simulink model "PowerSplitDriveUnitBasic_test_harness"  (R2020b)
settings: Solver=VariableStepAuto  StartTime=0.0  StopTime=t_end  RelTol=1e-3  AbsTol=1e-3
PreLoadFcn:
  | PowerSplitDriveUnitBasic_setup
undefined symbols (not defined in the file or in its folder): testharness
libraries: fl_lib x1, nesl_utility x1, EVComponents_utility_lib x1
settings Model: Creator=isaacito  LastModifiedBy=isaacito
settings SolverCC: AutoScaleAbsTol=off
settings DataIOCC: DSMLogging=off  InspectSignalLogs=on
settings SimscapeCC: SimscapeLogType=all  SimscapeLogSimulationStatistics=on  SimscapeLogLimitData=off

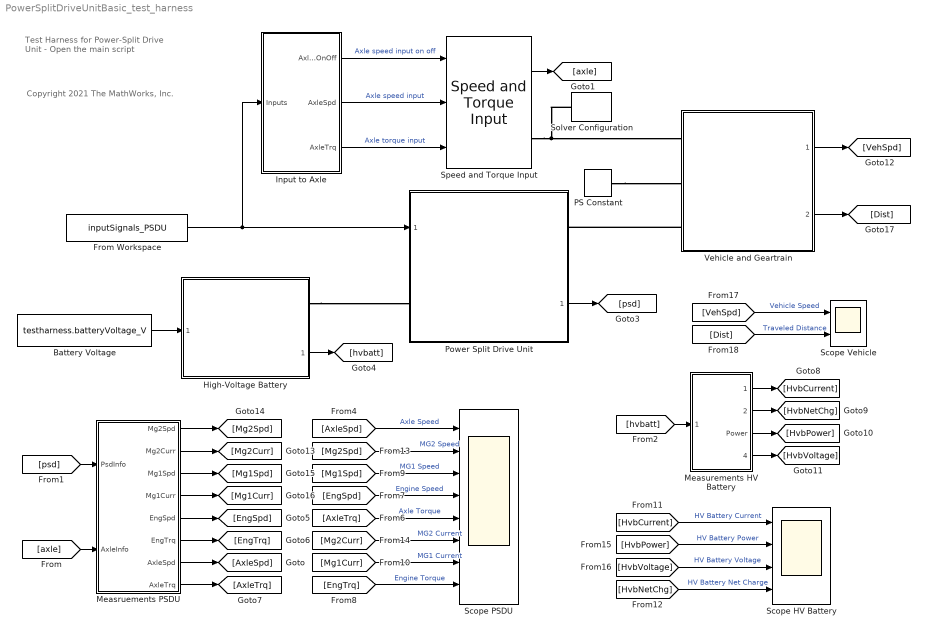
== system PowerSplitDriveUnitBasic_test_harness ==
  note: Copyright 2021 The MathWorks, Inc.
  note: Test Harness for
      | Power-Split Drive Unit
      | - Open the main script
  Battery Voltage : Constant  Value=testharness.batteryVoltage_V
  From Workspace : FromWorkspace  VariableName=inputSignals_PSDU  OutDataTypeStr=Bus: inputBus_PSDU  Interpolate=off  OutputAfterFinalValue=Holding final value
      settings: AttributesFormatString=%<OutDataTypeStr>
  High-Voltage Battery : Subsystem  ReferencedSubsystem=BatteryForTest_refsub
      settings: PortSchema="{\"entries\":[{\"content\":{\"sides\":[{\"content\":{\"connectorIds\":[\"In1\"]},\"type\":\"ConnectorPlacement.EquallySpacedRectSide\",\"uuid\":\"6ec42dc2-af13-403d-bb44-bbfe17049ebb\"},{\"content\":{\"connectorIds\":[\"RConn1\",\"Out1\"],\"side\":\"RIGHT\"},\"type\":\"ConnectorPlacement.EquallySpacedRectSide\",\"uuid\":\"18b43a22-b216-415c-b9ff-5dd426481655\"},{\"content\":{\"connectorIds\":[],\"side\":\"TOP\"},\"type\":\"ConnectorPlacement.EquallySpacedRectSide\",\"uuid\":\"9ddf6635-2c27-427a-8c83-df626a0e9ed3\"},{\"content\":{\"connectorIds\":[],\"side\":\"HIDDEN\"},\"type\":\"ConnectorPlacement.EquallySpacedRectSide\",\"uuid\":\"332981be-c8a8-46f3-86be-153015cc7779\"}]},\"type\":\"ConnectorPlacement.EquallySpacedConnector\",\"uuid\":\"0a64d723-305c-452f-a915-e14881ea19f7\"}],\"packageUris\":[\"http://schema.mathworks.com/mf0/Connector/R2020b\"],\"version\":\"1.0\"}"
  Input to Axle : Subsystem
  Measruements PSDU : Subsystem
  Measurements HV Battery : Subsystem
  PS Constant : fl_lib/Physical Signals/Sources/PS Constant  constant=0 N
      settings: AttributesFormatString=%<constant> [%<constant_unit>]
  Power Split Drive Unit : Subsystem  ReferencedSubsystem=PowerSplitDriveUnitBasic_refsub
      settings: PortSchema="{\"entries\":[{\"content\":{\"sides\":[{\"content\":{\"connectorIds\":[\"In1\",\"LConn1\"]},\"type\":\"ConnectorPlacement.EquallySpacedRectSide\",\"uuid\":\"ac3719a4-f5ca-49c1-b88d-60ddfcbc9c3c\"},{\"content\":{\"connectorIds\":[\"RConn1\",\"Out1\"],\"side\":\"RIGHT\"},\"type\":\"ConnectorPlacement.EquallySpacedRectSide\",\"uuid\":\"02c1cdca-c4bc-4e36-8da7-b9fd13165580\"},{\"content\":{\"connectorIds\":[],\"side\":\"TOP\"},\"type\":\"ConnectorPlacement.EquallySpacedRectSide\",\"uuid\":\"9a293679-982e-42e0-b445-a53b2f9deeb2\"},{\"content\":{\"connectorIds\":[],\"side\":\"HIDDEN\"},\"type\":\"ConnectorPlacement.EquallySpacedRectSide\",\"uuid\":\"92624000-5028-4c46-b75d-fdf82f03c691\"}]},\"type\":\"ConnectorPlacement.EquallySpacedConnector\",\"uuid\":\"49b414d9-6436-4fd3-904c-291d56adec0c\"}],\"packageUris\":[\"http://schema.mathworks.com/mf0/Connector/R2020b\"],\"version\":\"1.0\"}"
  Scope HV Battery : Scope  NumInputPorts=4
  Scope PSDU : Scope  NumInputPorts=8
  Scope Vehicle : Scope  NumInputPorts=2
  Solver Configuration : nesl_utility/Solver Configuration  PhysicalDomain=network_engine_domain  SubClassName=solver  LeftPortType=input  RightPortType=generic  Tones=[]  Harmonics=[]  SimulateNoise=off  Profile=off  UseLocalSampling=off  EnableSwitchedLinearOptims=on  FrequencyDomain=off  UseCCode=off  RelTol=0.001  AbsTol=1e-06  MinStep=1e-09  ToWorkspace=off  RevertToSquareIcSolve=off  NumHomotopyIterations=100  PhasorMode=off  PhasorModeNumHarmonics=1  DoDC=off  ResidualTolerance=1e-09  UseLocalSolver=off  LocalSolverChoice=NE_BACKWARD_EULER_ADVANCER  LocalSolverSampleTime=0.001  DoFixedCost=off  MaxNonlinIter=3  MaxModeIter=2  ComputeImpulses=off  ImpulseIterations=2  LinearAlgebra=auto  EquationFormulation=NE_TIME_EF  DelaysMemoryBudget=1024  AutomaticFiltering=on  FilteringTimeConstant=0.001  PartitionStorageMethod=AS_NEEDED  PartitionMemoryBudget=1024  PartitionMethod=ROBUST
      settings: AttributesFormatString=Local sover: %<UseLocalSolver>
  Speed and Torque Input : EVComponents_utility_lib/Speed and Torque Input  t_friction=10000  t_locked=10000  w_tol=0.001  initial_state_locked=sdl.enum.initial_lock.unlocked
  Vehicle and Geartrain : Subsystem  ReferencedSubsystem=VehicleForTest_refsub
      settings: PortSchema="{\"entries\":[{\"content\":{\"sides\":[{\"content\":{\"connectorIds\":[\"LConn1\",\"LConn3\",\"LConn2\"]},\"type\":\"ConnectorPlacement.EquallySpacedRectSide\",\"uuid\":\"c975ecd5-3624-4c19-9a80-acedd8bc41a3\"},{\"content\":{\"connectorIds\":[\"Out1\",\"Out2\"],\"side\":\"RIGHT\"},\"type\":\"ConnectorPlacement.EquallySpacedRectSide\",\"uuid\":\"910143c3-3967-4448-a629-d08cf6777789\"},{\"content\":{\"connectorIds\":[],\"side\":\"TOP\"},\"type\":\"ConnectorPlacement.EquallySpacedRectSide\",\"uuid\":\"7a417a30-364f-4b70-8ba2-82e05b7f8ad5\"},{\"content\":{\"connectorIds\":[],\"side\":\"HIDDEN\"},\"type\":\"ConnectorPlacement.EquallySpacedRectSide\",\"uuid\":\"66b5b01a-20fa-4f6a-8c11-38a64c540bf5\"}]},\"type\":\"ConnectorPlacement.EquallySpacedConnector\",\"uuid\":\"d97c4709-181f-4fdd-bd6d-fe96f1a8d0ed\"}],\"packageUris\":[\"http://schema.mathworks.com/mf0/Connector/R2020b\"],\"version\":\"1.0\"}"
  wires:
  Battery Voltage/1 -> High-Voltage Battery/1
  Input to Axle/2(AxleSpd) -> Speed and Torque Input/2  "Axle speed input"
  Input to Axle/1(AxleSpd_OnOff) -> Speed and Torque Input/1  "Axle speed input on off"
  Input to Axle/3(AxleTrq) -> Speed and Torque Input/3  "Axle torque input"
  From Workspace/1 -> Power Split Drive Unit/1, Input to Axle/1(Inputs)
  Speed and Torque Input/1 -> [axle]
  Power Split Drive Unit/1 -> [psd]
  [axle] -> Measruements PSDU/2(AxleInfo)
  [psd] -> Measruements PSDU/1(PsdInfo)
  [EngTrq] -> Scope PSDU/8  "Engine Torque"
  [Mg1Curr] -> Scope PSDU/7  "MG1 Current"
  [EngSpd] -> Scope PSDU/4  "Engine Speed"
  [Mg1Spd] -> Scope PSDU/3  "MG1 Speed"
  [AxleSpd] -> Scope PSDU/1  "Axle Speed"
  [AxleTrq] -> Scope PSDU/5  "Axle Torque"
  [Mg2Curr] -> Scope PSDU/6  "MG2 Current"
  [Mg2Spd] -> Scope PSDU/2  "MG2 Speed"
  Measruements PSDU/1(Mg2Spd) -> [Mg2Spd]
  Measruements PSDU/2(Mg2Curr) -> [Mg2Curr]
  Measruements PSDU/3(Mg1Spd) -> [Mg1Spd]
  Measruements PSDU/4(Mg1Curr) -> [Mg1Curr]
  Measruements PSDU/5(EngSpd) -> [EngSpd]
  Measruements PSDU/6(EngTrq) -> [EngTrq]
  Measruements PSDU/7(AxleSpd) -> [AxleSpd]
  Measruements PSDU/8(AxleTrq) -> [AxleTrq]
  [hvbatt] -> Measurements HV Battery/1(HVBatt)
  [HvbPower] -> Scope HV Battery/2  "HV Battery Power"
  [HvbNetChg] -> Scope HV Battery/4  "HV Battery Net Charge"
  [HvbVoltage] -> Scope HV Battery/3  "HV Battery Voltage"
  [HvbCurrent] -> Scope HV Battery/1  "HV Battery Current"
  Measurements HV Battery/1(Current) -> [HvbCurrent]
  Measurements HV Battery/2(NetChg) -> [HvbNetChg]
  Measurements HV Battery/3(Power) -> [HvbPower]
  Measurements HV Battery/4(Voltage) -> [HvbVoltage]
  Vehicle and Geartrain/1 -> [VehSpd]
  Vehicle and Geartrain/2 -> [Dist]
  [VehSpd] -> Scope Vehicle/1  "Vehicle Speed"
  [Dist] -> Scope Vehicle/2  "Traveled Distance"
  High-Voltage Battery/1 -> [hvbatt]
  connections:
  Vehicle and Geartrain/LConn2 -- Power Split Drive Unit/RConn1
  Speed and Torque Input/RConn1 -- Vehicle and Geartrain/LConn1 -- Solver Configuration/RConn1
  PS Constant/RConn1 -- Vehicle and Geartrain/LConn3
  High-Voltage Battery/RConn1 -- Power Split Drive Unit/LConn1

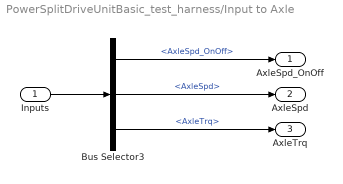
== system PowerSplitDriveUnitBasic_test_harness/Input to Axle ==
  Inputs : Inport
  Bus Selector3 : BusSelector  OutputSignals=AxleSpd_OnOff,AxleSpd,AxleTrq
  AxleSpd_OnOff : Outport
  AxleSpd : Outport  Port=2
  AxleTrq : Outport  Port=3
  wires:
  Bus Selector3/2 -> AxleSpd/1  "<AxleSpd>"
  Inputs/1 -> Bus Selector3/1
  Bus Selector3/1 -> AxleSpd_OnOff/1  "<AxleSpd_OnOff>"
  Bus Selector3/3 -> AxleTrq/1  "<AxleTrq>"

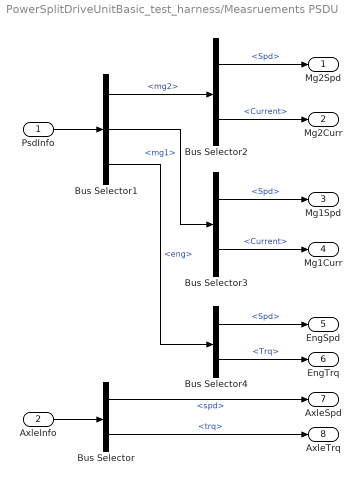
== system PowerSplitDriveUnitBasic_test_harness/Measruements PSDU ==
  PsdInfo : Inport
  AxleInfo : Inport  Port=2
  Bus Selector : BusSelector  OutputSignals=spd,trq
  Bus Selector1 : BusSelector  OutputSignals=mg2,mg1,eng
  Bus Selector2 : BusSelector  OutputSignals=Spd,Current
  Bus Selector3 : BusSelector  OutputSignals=Spd,Current
  Bus Selector4 : BusSelector  OutputSignals=Spd,Trq
  Mg2Spd : Outport
  Mg2Curr : Outport  Port=2
  Mg1Spd : Outport  Port=3
  Mg1Curr : Outport  Port=4
  EngSpd : Outport  Port=5
  EngTrq : Outport  Port=6
  AxleSpd : Outport  Port=7
  AxleTrq : Outport  Port=8
  wires:
  AxleInfo/1 -> Bus Selector/1
  PsdInfo/1 -> Bus Selector1/1
  Bus Selector1/1 -> Bus Selector2/1  "<mg2>"
  Bus Selector1/2 -> Bus Selector3/1  "<mg1>"
  Bus Selector1/3 -> Bus Selector4/1  "<eng>"
  Bus Selector2/1 -> Mg2Spd/1  "<Spd>"
  Bus Selector2/2 -> Mg2Curr/1  "<Current>"
  Bus Selector3/1 -> Mg1Spd/1  "<Spd>"
  Bus Selector3/2 -> Mg1Curr/1  "<Current>"
  Bus Selector4/1 -> EngSpd/1  "<Spd>"
  Bus Selector4/2 -> EngTrq/1  "<Trq>"
  Bus Selector/1 -> AxleSpd/1  "<spd>"
  Bus Selector/2 -> AxleTrq/1  "<trq>"

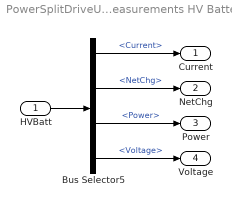
== system PowerSplitDriveUnitBasic_test_harness/Measurements HV Battery ==
  HVBatt : Inport
  Bus Selector5 : BusSelector  OutputSignals=Current,NetChg,Power,Voltage
  Current : Outport
  NetChg : Outport  Port=2
  Power : Outport  Port=3
  Voltage : Outport  Port=4
  wires:
  Bus Selector5/4 -> Voltage/1  "<Voltage>"
  Bus Selector5/2 -> NetChg/1  "<NetChg>"
  Bus Selector5/3 -> Power/1  "<Power>"
  HVBatt/1 -> Bus Selector5/1
  Bus Selector5/1 -> Current/1  "<Current>"
